simulink model "PV_MPPT (1)"  (R2025b)
settings: Solver=VariableStepAuto  StartTime=0.0  StopTime=160  FixedStep=0.01  MaxStep=1e-3  MinStep=1e-12  RelTol=1e-2
undefined symbols (not defined in the file): DiscIntNeverNeededParam
libraries: simulink x3, slpidlib x2

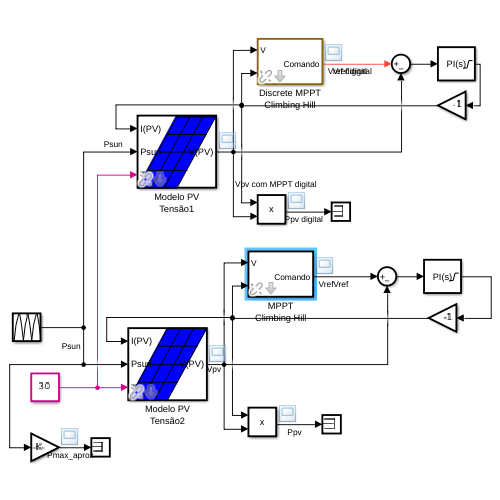
[thumbnail: Simulink's stored preview of the top-level diagram]
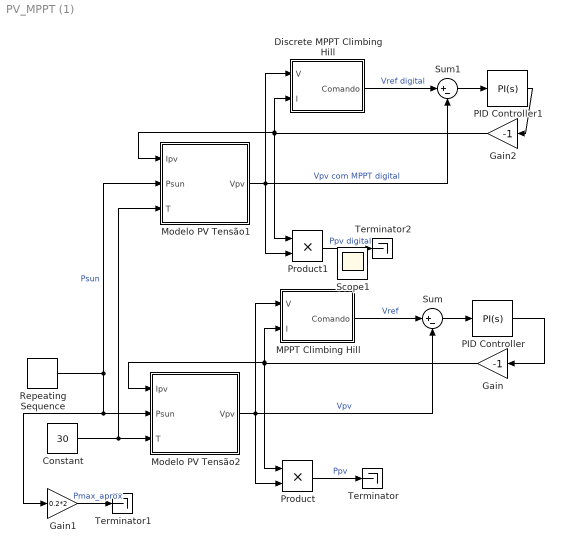
== system PV_MPPT (1) ==
  Constant : Constant  Value=30
  Discrete MPPT Climbing Hill : Subsystem  AncestorBlock=AvgModels/MPPT/MPPT Climbing Hill  mask(MPPT Hill Climbing){Ts=0.01, Passo=2, limsup=30*2, liminf=10*2, Inicial=25*2, sentido=Direto}
      mask prompts: Ts "Tempo de amostragem:"; Passo "Passo de variação"; limsup "Limite superior da saída:"; liminf "Limite inferior da saída:"; Inicial "Valor inicial:"; sentido "Direção do Comando:"
      mask help:
      | Algoritmo de rastreamento do ponto de máxima potência (MPPT).
      | Princípio da escalada ou Perturbe and Observe (P&O).
  Gain : Gain  Gain=-1
  Gain1 : Gain  Gain=0.2*2
  Gain2 : Gain  Gain=-1
  MPPT Climbing Hill : Subsystem  AncestorBlock=AvgModels/MPPT/MPPT Climbing Hill  mask(MPPT Hill Climbing){fb=100, Passo=2, limsup=30*2, liminf=15*2, Inicial=25*2, sentido=Direto}
      mask prompts: fb "Filtro de derivação:"; Passo "Passo de variação"; limsup "Limite superior da saída:"; liminf "Limite inferior da saída:"; Inicial "Valor inicial:"; sentido "Direção do comando:"
      mask help:
      | Algoritmo de rastreamento do ponto de máxima potência (MPPT).
      | Princípio da escalada ou Perturbe and Observe (P&O).
  Modelo PV Tensão1 : Subsystem  AncestorBlock=AvgModels/Fontes/Modelo PV Tensão  mask(Modelo PV de tensão){Ns=54, Voc=0.6093, Isc=8.21, Rs=0.005, Rp=7, Ms=2, Mp=1, Tr=273 + 25, a=3.18e-3, n=1.2, k=1.38e-23, q=1.60e-19, EG=1.1, tau=0.1, Psun=1000, Animar=off}
      mask prompts: Ns "Número de células"; Voc "Tensão de circuito aberto (Voc por célula)"; Isc "Corrente de curto-circuito (Isc)"; Rs "Resistência série da célula"; Rp "Resistência paralela da célula"; Ms "Módulos em Série"; Mp "Módulos em Paralelo"; Tr "Temperatura Ambiente (K)"; a "Coeficiente de temperatura de Isc:"; n "Fator de qualidade da junção p-n:"; k "Constante de Boltzmann:"; q "Carga do elétron:"; EG "Energia da banda proibida:"; tau "Contante de tempo (s):"; Psun "Irradiação de teste (W/m2):"; Animar "Animar em execução?"
      mask help:
      | Este é um modelo de tensão para painéis fotovoltaicos (sozinhos ou em arranjo).
      |
      | Fornece a tensão esperada de acordo com a corrente, a densidade de potência do sol e a temperatura ambiente.
      |
      | I(PV) é a corrente do arranjo fotovoltaico em Amperes.
      | Psun é a densidade de potência do sol em W/m2.
      | T é a temperatura ambiente em ºC.
      |
      | V(PV) é a tensão do arranjo fotovoltaico em Amperes.
      mask DialogControl ParameterGroupVar Prompt: Parâmetros
      mask DialogControl Container4 Prompt: Por módulo
      mask DialogControl Container6 Prompt: Local
      mask DialogControl Container5 Prompt: Constantes
      mask DialogControl Container9 Prompt: Verificação da curva.
      mask DialogControl Control2 Prompt: Verificar Curvas
      mask DialogControl Control2 Callback:
      | Psun = str2num(get_param(gcbh,'Psun'));
      | Tr = str2num(get_param(gcbh,'Tr'));
      | Voc = str2num(get_param(gcbh,'Voc'));
      | Isc = str2num(get_param(gcbh,'Isc'));
      | Rp = str2num(get_param(gcbh,'Rp'));
      | Rs = str2num(get_param(gcbh,'Rs'));
      | Ns = str2num(get_param(gcbh,'Ns'));
      | alpha = str2num(get_param(gcbh,'a'));
      | encontrapmax(Psun,Tr-273,Voc,Isc,Rp,Rs,Ns,alpha);
      mask Display:
      | % desenho detalhado
      | patch([0 .5 1 .5],[0 1 1 0],[0 0 1]);
      | plot([0 0.5],[0 1])
      | plot([0.5/3 0.5+0.5/3],[0 1])
      | plot([0.5/3 0.5+0.5/3]+0.5/3,[0 1])
      | plot([0.5 1],[0 1])
      | 
      | plot([0 0.5],[0 0])
      | plot([0 0.5]+0.125,[0 0]+0.25)
      | plot([0 0.5]+0.25,[0 0]+0.5)
      | plot([0 0.5]+0.25+0.125,[0 0]+0.75)
      | plot([0.5 1],[1 1])
      | 
      | 
      | port_label('output',1,'V(PV)');
      | 
      | port_label('input',1,'I(PV)');
      | port_label('input',2,'Psun');
      | port_label('input',3,'T');
  Modelo PV Tensão2 : Subsystem  AncestorBlock=AvgModels/Fontes/Modelo PV Tensão  mask(Modelo PV de tensão){Ns=54, Voc=0.6093, Isc=8.21, Rs=0.005, Rp=7, Ms=2, Mp=1, Tr=273 + 25, a=3.18e-3, n=1.2, k=1.38e-23, q=1.60e-19, EG=1.1, tau=0.1, Psun=1000, Animar=off}
      mask prompts: Ns "Número de células"; Voc "Tensão de circuito aberto (Voc por célula)"; Isc "Corrente de curto-circuito (Isc)"; Rs "Resistência série da célula"; Rp "Resistência paralela da célula"; Ms "Módulos em Série"; Mp "Módulos em Paralelo"; Tr "Temperatura Ambiente (K)"; a "Coeficiente de temperatura de Isc:"; n "Fator de qualidade da junção p-n:"; k "Constante de Boltzmann:"; q "Carga do elétron:"; EG "Energia da banda proibida:"; tau "Contante de tempo (s):"; Psun "Irradiação de teste (W/m2):"; Animar "Animar em execução?"
      mask help:
      | Este é um modelo de tensão para painéis fotovoltaicos (sozinhos ou em arranjo).
      |
      | Fornece a tensão esperada de acordo com a corrente, a densidade de potência do sol e a temperatura ambiente.
      |
      | I(PV) é a corrente do arranjo fotovoltaico em Amperes.
      | Psun é a densidade de potência do sol em W/m2.
      | T é a temperatura ambiente em ºC.
      |
      | V(PV) é a tensão do arranjo fotovoltaico em Amperes.
      mask DialogControl ParameterGroupVar Prompt: Parâmetros
      mask DialogControl Container4 Prompt: Por módulo
      mask DialogControl Container6 Prompt: Local
      mask DialogControl Container5 Prompt: Constantes
      mask DialogControl Container9 Prompt: Verificação da curva.
      mask DialogControl Control2 Prompt: Verificar Curvas
      mask DialogControl Control2 Callback:
      | Psun = str2num(get_param(gcbh,'Psun'));
      | Tr = str2num(get_param(gcbh,'Tr'));
      | Voc = str2num(get_param(gcbh,'Voc'));
      | Isc = str2num(get_param(gcbh,'Isc'));
      | Rp = str2num(get_param(gcbh,'Rp'));
      | Rs = str2num(get_param(gcbh,'Rs'));
      | Ns = str2num(get_param(gcbh,'Ns'));
      | alpha = str2num(get_param(gcbh,'a'));
      | encontrapmax(Psun,Tr-273,Voc,Isc,Rp,Rs,Ns,alpha);
      mask Display:
      | % desenho detalhado
      | patch([0 .5 1 .5],[0 1 1 0],[0 0 1]);
      | plot([0 0.5],[0 1])
      | plot([0.5/3 0.5+0.5/3],[0 1])
      | plot([0.5/3 0.5+0.5/3]+0.5/3,[0 1])
      | plot([0.5 1],[0 1])
      | 
      | plot([0 0.5],[0 0])
      | plot([0 0.5]+0.125,[0 0]+0.25)
      | plot([0 0.5]+0.25,[0 0]+0.5)
      | plot([0 0.5]+0.25+0.125,[0 0]+0.75)
      | plot([0.5 1],[1 1])
      | 
      | 
      | port_label('output',1,'V(PV)');
      | 
      | port_label('input',1,'I(PV)');
      | port_label('input',2,'Psun');
      | port_label('input',3,'T');
  PID Controller : slpidlib/PID Controller  Controller=PI  Form=Parallel  TimeDomain=Continuous-time  UseExternalTs=off  SampleTime=-1  IntegratorMethod=Forward Euler  FilterMethod=Forward Euler  ControllerParametersSource=internal  P=1  I=1  UseKiTs=off  D=0  UseExternalDerivativeSource=off  N=100  UseFilter=on  TunerSelectOption=Transfer Function Based (PID Tuner App)  InitialConditionSource=internal  InitialConditionForIntegrator=-1  InitialConditionForFilter=0  DifferentiatorICPrevScaledInput=0  ExternalReset=none  TrackingMode=off  Kt=1  LimitOutput=on  SatLimitsSource=internal  UpperSaturationLimit=-0.5  LowerSaturationLimit=-8  LinearizeAsGain=on  AntiWindupMode=none  Kb=1  LimitIntegrator=off  UpperIntegratorSaturationLimit=inf  LowerIntegratorSaturationLimit=-inf  POutMin=[]  POutMax=[]  IOutMin=[]  IOutMax=[]  DOutMin=[]  DOutMax=[]  NOutMin=[]  NOutMax=[]  SumOutMin=[]  SumOutMax=[]  SaturationOutMin=[]  SaturationOutMax=[]  PParamMin=[]  PParamMax=[]  IParamMin=[]  IParamMax=[]  DParamMin=[]  DParamMax=[]  NParamMin=[]  NParamMax=[]  KbParamMin=[]  KbParamMax=[]  KtParamMin=[]  KtParamMax=[]  KbOutMin=[]  KbOutMax=[]  KtOutMin=[]  KtOutMax=[]  IntegratorOutMin=[]  IntegratorOutMax=[]  FilterOutMin=[]  FilterOutMax=[]  SumI1OutMin=[]  SumI1OutMax=[]  SumI2OutMin=[]  SumI2OutMax=[]  SumI3OutMin=[]  SumI3OutMax=[]  SumI4OutMin=[]  SumI4OutMax=[]  SumDOutMin=[]  SumDOutMax=[]  DifferentiatorOutMin=[]  DifferentiatorOutMax=[]  FilterDiffOutCoefMin=[]  FilterDiffOutCoefMax=[]  ReciprocalOutMin=[]  ReciprocalOutMax=[]  SumDenOutMin=[]  SumDenOutMax=[]  SumNumOutMin=[]  SumNumOutMax=[]  DivideOutMin=[]  DivideOutMax=[]  UdiffTsProdOutMin=[]  UdiffTsProdOutMax=[]  NTsProdOutMin=[]  NTsProdOutMax=[]  UintegralTsProdOutMin=[]  UintegralTsProdOutMax=[]  UngainTsProdOutMin=[]  UngainTsProdOutMax=[]  ClampingZeroOutDataTypeStr=Inherit: Inherit via back propagation  ClampingZeroOutMin=[]  ClampingZeroOutMax=[]  FilterDenConstantOutDataTypeStr=Inherit: Inherit via back propagation  FilterDenConstantOutMin=[]  FilterDenConstantOutMax=[]  PCopyOutDataTypeStr=Inherit: Inherit via back propagation  PCopyOutMin=[]  PCopyOutMax=[]  NCopyOutDataTypeStr=Inherit: Inherit via back propagation  NCopyOutMin=[]  NCopyOutMax=[]  IntegratorContinuousStateAttributes=''  IntegratorStateMustResolveToSignalObject=off  IntegratorRTWStateStorageClass=Auto  FilterContinuousStateAttributes=''  FilterStateMustResolveToSignalObject=off  FilterRTWStateStorageClass=Auto  ParallelPVariant=InternalParameters  IdealPVariant=Disabled  IVariant=InternalParameters  DVariant=Disabled  IntegratorVariant=Continuous  SatVariant=Enabled  AWVariant=Passthrough  PCopyVariant=Disabled  TRVariant=Disabled  FdbkBlocksVariant=Forward  IdealPFdbkVariant=Disabled  SatFdbkVariant=Disabled  DerivativeFilterVariant=Disabled  NVariant=Disabled  NCopyVariant=Disabled_SignalSpec  FilterICVariant=Disabled  IntegratorICVariant=InternalICs  ExternalResetVariant=Disabled  TRSumVariant=Passthrough  SumFdbkVariant=Disabled  SumVariant=Sum_PI  TsampFilterVariant=InternalTs  TsampNgainVariant=Passthrough  TsampIntegralVariant=Disabled_SignalSpec  ExternalSaturationOutDataTypeStr=Inherit: Same as second input  DerivativeSourceVariant=Disabled  PreIntVariant=InternalPreInt
  PID Controller1 : slpidlib/PID Controller  Controller=PI  Form=Parallel  TimeDomain=Continuous-time  UseExternalTs=off  SampleTime=-1  IntegratorMethod=Forward Euler  FilterMethod=Forward Euler  ControllerParametersSource=internal  P=1  I=1  UseKiTs=off  D=0  UseExternalDerivativeSource=off  N=100  UseFilter=on  TunerSelectOption=Transfer Function Based (PID Tuner App)  InitialConditionSource=internal  InitialConditionForIntegrator=-1  InitialConditionForFilter=0  DifferentiatorICPrevScaledInput=0  ExternalReset=none  TrackingMode=off  Kt=1  LimitOutput=on  SatLimitsSource=internal  UpperSaturationLimit=-0.5  LowerSaturationLimit=-8  LinearizeAsGain=on  AntiWindupMode=clamping  Kb=1  LimitIntegrator=off  UpperIntegratorSaturationLimit=inf  LowerIntegratorSaturationLimit=-inf  POutMin=[]  POutMax=[]  IOutMin=[]  IOutMax=[]  DOutMin=[]  DOutMax=[]  NOutMin=[]  NOutMax=[]  SumOutMin=[]  SumOutMax=[]  SaturationOutMin=[]  SaturationOutMax=[]  PParamMin=[]  PParamMax=[]  IParamMin=[]  IParamMax=[]  DParamMin=[]  DParamMax=[]  NParamMin=[]  NParamMax=[]  KbParamMin=[]  KbParamMax=[]  KtParamMin=[]  KtParamMax=[]  KbOutMin=[]  KbOutMax=[]  KtOutMin=[]  KtOutMax=[]  IntegratorOutMin=[]  IntegratorOutMax=[]  FilterOutMin=[]  FilterOutMax=[]  SumI1OutMin=[]  SumI1OutMax=[]  SumI2OutMin=[]  SumI2OutMax=[]  SumI3OutMin=[]  SumI3OutMax=[]  SumI4OutMin=[]  SumI4OutMax=[]  SumDOutMin=[]  SumDOutMax=[]  DifferentiatorOutMin=[]  DifferentiatorOutMax=[]  FilterDiffOutCoefMin=[]  FilterDiffOutCoefMax=[]  ReciprocalOutMin=[]  ReciprocalOutMax=[]  SumDenOutMin=[]  SumDenOutMax=[]  SumNumOutMin=[]  SumNumOutMax=[]  DivideOutMin=[]  DivideOutMax=[]  UdiffTsProdOutMin=[]  UdiffTsProdOutMax=[]  NTsProdOutMin=[]  NTsProdOutMax=[]  UintegralTsProdOutMin=[]  UintegralTsProdOutMax=[]  UngainTsProdOutMin=[]  UngainTsProdOutMax=[]  ClampingZeroOutDataTypeStr=Inherit: Inherit via back propagation  ClampingZeroOutMin=[]  ClampingZeroOutMax=[]  FilterDenConstantOutDataTypeStr=Inherit: Inherit via back propagation  FilterDenConstantOutMin=[]  FilterDenConstantOutMax=[]  PCopyOutDataTypeStr=Inherit: Inherit via back propagation  PCopyOutMin=[]  PCopyOutMax=[]  NCopyOutDataTypeStr=Inherit: Inherit via back propagation  NCopyOutMin=[]  NCopyOutMax=[]  IntegratorContinuousStateAttributes=''  IntegratorStateMustResolveToSignalObject=off  IntegratorRTWStateStorageClass=Auto  FilterContinuousStateAttributes=''  FilterStateMustResolveToSignalObject=off  FilterRTWStateStorageClass=Auto  ParallelPVariant=InternalParameters  IdealPVariant=Disabled  IVariant=InternalParameters  DVariant=Disabled  IntegratorVariant=Continuous  SatVariant=Enabled  AWVariant=ContClampingParallel  PCopyVariant=Disabled  TRVariant=Disabled  FdbkBlocksVariant=Forward  IdealPFdbkVariant=Disabled  SatFdbkVariant=Disabled  DerivativeFilterVariant=Disabled  NVariant=Disabled  NCopyVariant=Disabled_SignalSpec  FilterICVariant=Disabled  IntegratorICVariant=InternalICs  ExternalResetVariant=Disabled  TRSumVariant=Passthrough  SumFdbkVariant=Disabled  SumVariant=Sum_PI  TsampFilterVariant=InternalTs  TsampNgainVariant=Passthrough  TsampIntegralVariant=Disabled_SignalSpec  ExternalSaturationOutDataTypeStr=Inherit: Same as second input  DerivativeSourceVariant=Disabled  PreIntVariant=InternalPreInt
  Product : Product
  Product1 : Product
  Repeating Sequence : simulink/Sources/Repeating Sequence  rep_seq_t=[0 2 4 5 6 8 10]*4  rep_seq_y=[1 5 7 8 8 5 1]*100
  Sum : Sum  Inputs=|+-
  Sum1 : Sum  Inputs=|+-
  Terminator : Terminator
  Terminator1 : Terminator
  Terminator2 : Terminator
  Scope1 : Scope
      settings: ActiveDisplayYMinimum=-7.8557532744699214  ActiveDisplayYMaximum=70.701779470229312
  wires:
  Modelo PV Tensão2/1(Vpv) -> Sum/2, Product/2, MPPT Climbing Hill/1(V)  "Vpv"
  Sum/1 -> PID Controller/1
  PID Controller/1 -> Gain/1
  Gain/1 -> Modelo PV Tensão2/1(Ipv), MPPT Climbing Hill/2(I), Product/1
  Product/1 -> Terminator/1  "Ppv"
  Gain1/1 -> Terminator1/1  "Pmax_aprox"
  MPPT Climbing Hill/1(Comando) -> Sum/1  "Vref"
  Discrete MPPT Climbing Hill/1(Comando) -> Sum1/1  "Vref digital"
  Product1/1 -> Terminator2/1  "Ppv digital"
  Gain2/1 -> Product1/1, Discrete MPPT Climbing Hill/2(I), Modelo PV Tensão1/1(Ipv)
  PID Controller1/1 -> Gain2/1
  Repeating Sequence/1 -> Modelo PV Tensão2/2(Psun), Gain1/1, Modelo PV Tensão1/2(Psun)  "Psun"
  Constant/1 -> Modelo PV Tensão2/3(T), Modelo PV Tensão1/3(T)
  Sum1/1 -> PID Controller1/1
  Modelo PV Tensão1/1(Vpv) -> Discrete MPPT Climbing Hill/1(V), Product1/2, Sum1/2  "Vpv com MPPT digital"

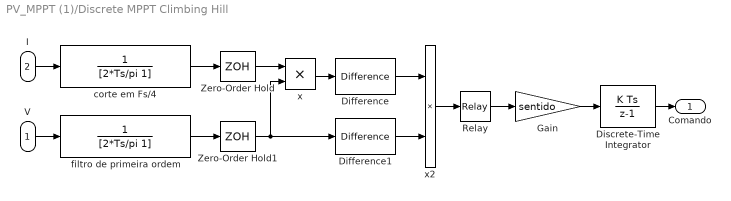
== system PV_MPPT (1)/Discrete MPPT Climbing Hill ==
  V : Inport
  I : Inport  Port=2
  Difference : simulink/Discrete/Difference  ICPrevInput=Ts  OutMin=[]  OutMax=[]  OutDataType=fixdt(1, 16)  OutScaling=2^-10  DoSatur=off
  Difference1 : simulink/Discrete/Difference  ICPrevInput=Ts  OutMin=[]  OutMax=[]  OutDataType=fixdt(1, 16)  OutScaling=2^-10  DoSatur=off
  Discrete-Time Integrator : DiscreteIntegrator  gainval=Passo  InitialCondition=Inicial  SampleTime=Ts  LimitOutput=on  UpperSaturationLimit=limsup  LowerSaturationLimit=liminf  ICPrevOutput=DiscIntNeverNeededParam  ICPrevScaledInput=DiscIntNeverNeededParam
  Gain : Gain  Gain=sentido
  Relay : Relay  OnSwitchValue=1  OffSwitchValue=-1  OffOutputValue=-1  ZeroCross=off
  Zero-Order Hold : ZeroOrderHold  SampleTime=Ts
  Zero-Order Hold1 : ZeroOrderHold  SampleTime=Ts
  corte em Fs/4 : TransferFcn  Denominator=[2*Ts/pi 1]
  filtro de primeira ordem : TransferFcn  Denominator=[2*Ts/pi 1]
  x : Product  RndMeth=Zero
  x2 : Product  RndMeth=Zero
  Comando : Outport
  wires:
  x/1 -> Difference/1
  Difference/1 -> x2/1
  Difference1/1 -> x2/2
  V/1 -> filtro de primeira ordem/1
  I/1 -> corte em Fs/4/1
  x2/1 -> Relay/1
  Relay/1 -> Gain/1
  Discrete-Time Integrator/1 -> Comando/1
  Zero-Order Hold/1 -> x/1
  Zero-Order Hold1/1 -> x/2, Difference1/1
  corte em Fs/4/1 -> Zero-Order Hold/1
  filtro de primeira ordem/1 -> Zero-Order Hold1/1
  Gain/1 -> Discrete-Time Integrator/1

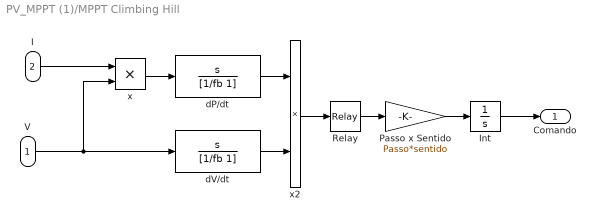
== system PV_MPPT (1)/MPPT Climbing Hill ==
  V : Inport
  I : Inport  Port=2
  Int : Integrator  InitialCondition=Inicial  LimitOutput=on  UpperSaturationLimit=limsup  LowerSaturationLimit=liminf
  Passo x Sentido : Gain  Gain=Passo*sentido
  Relay : Relay  OnSwitchValue=1  OffSwitchValue=-1  OffOutputValue=-1  ZeroCross=off
  dP/dt : TransferFcn  Numerator=[1 0]  Denominator=[1/fb 1]
  dV/dt : TransferFcn  Numerator=[1 0]  Denominator=[1/fb 1]
  x : Product  RndMeth=Zero
  x2 : Product  RndMeth=Zero
  Comando : Outport
  wires:
  Int/1 -> Comando/1
  x2/1 -> Relay/1
  I/1 -> x/1
  V/1 -> x/2, dV/dt/1
  dV/dt/1 -> x2/2
  dP/dt/1 -> x2/1
  x/1 -> dP/dt/1
  Relay/1 -> Passo x Sentido/1
  Passo x Sentido/1 -> Int/1

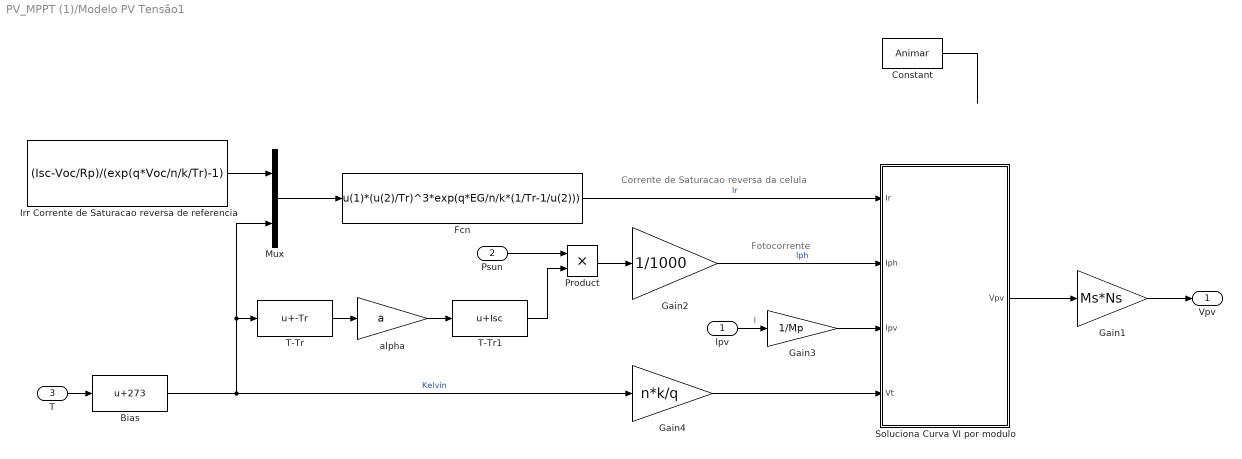
== system PV_MPPT (1)/Modelo PV Tensão1 ==
  note: Fotocorrente
  note: Corrente de Saturacao reversa da celula
  Ipv : Inport
  Psun : Inport  Port=2
  T : Inport  Port=3
  Bias : Bias  Bias=273  SaturateOnIntegerOverflow=off
  Constant : Constant  Value=Animar
  Fcn : Fcn  Expr=u(1)*(u(2)/Tr)^3*exp(q*EG/n/k*(1/Tr-1/u(2)))
  Gain1 : Gain  Gain=Ms*Ns
  Gain2 : Gain  Gain=1/1000
  Gain3 : Gain  Gain=1/Mp
  Gain4 : Gain  Gain=n*k/q
  Irr Corrente de Saturacao reversa de referencia : Constant  Value=(Isc-Voc/Rp)/(exp(q*Voc/n/k/Tr)-1)
  Mux : Mux  Inputs=2
  Product : Product
  Soluciona Curva VI por modulo : Subsystem
  T-Tr : Bias  Bias=-Tr  SaturateOnIntegerOverflow=off
  T-Tr1 : Bias  Bias=Isc  SaturateOnIntegerOverflow=off
  alpha : Gain  Gain=a
  Vpv : Outport
  wires:
  Irr Corrente de Saturacao reversa de referencia/1 -> Mux/1
  Mux/1 -> Fcn/1
  Psun/1 -> Product/1
  T-Tr1/1 -> Product/2
  Product/1 -> Gain2/1
  alpha/1 -> T-Tr1/1
  T-Tr/1 -> alpha/1
  T/1 -> Bias/1
  Bias/1 -> T-Tr/1, Mux/2, Gain4/1  "Kelvin"
  Gain4/1 -> Soluciona Curva VI por modulo/4(Vt)
  Fcn/1 -> Soluciona Curva VI por modulo/1(Ir)  "Ir"
  Gain2/1 -> Soluciona Curva VI por modulo/2(Iph)  "Iph"
  Ipv/1 -> Gain3/1  "I"
  Soluciona Curva VI por modulo/1(Vpv) -> Gain1/1
  Gain1/1 -> Vpv/1
  Gain3/1 -> Soluciona Curva VI por modulo/3(Ipv)
  Constant/1 -> ?

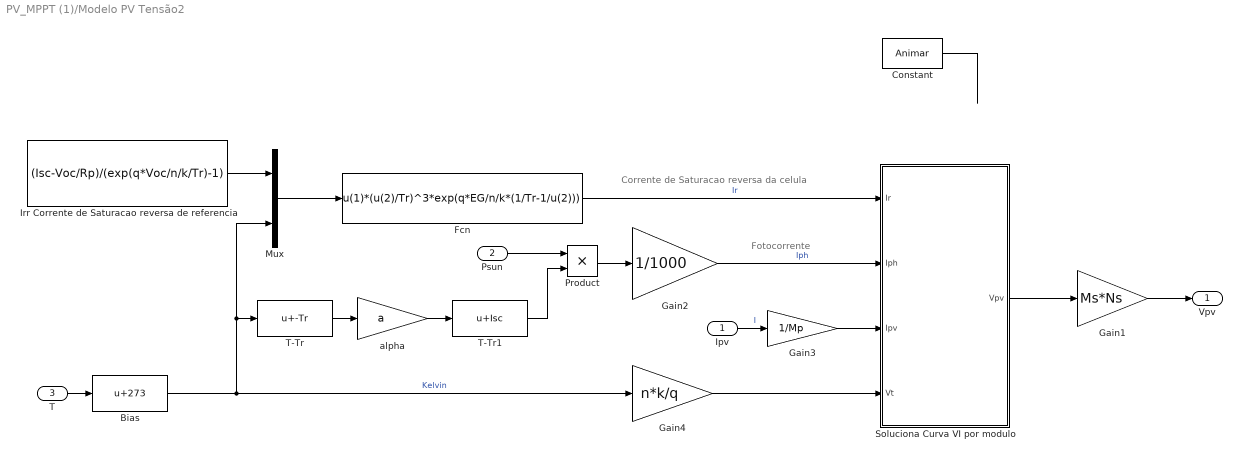
== system PV_MPPT (1)/Modelo PV Tensão2 ==
  note: Corrente de Saturacao reversa da celula
  note: Fotocorrente
  Ipv : Inport
  Psun : Inport  Port=2
  T : Inport  Port=3
  Bias : Bias  Bias=273  SaturateOnIntegerOverflow=off
  Constant : Constant  Value=Animar
  Fcn : Fcn  Expr=u(1)*(u(2)/Tr)^3*exp(q*EG/n/k*(1/Tr-1/u(2)))
  Gain1 : Gain  Gain=Ms*Ns
  Gain2 : Gain  Gain=1/1000
  Gain3 : Gain  Gain=1/Mp
  Gain4 : Gain  Gain=n*k/q
  Irr Corrente de Saturacao reversa de referencia : Constant  Value=(Isc-Voc/Rp)/(exp(q*Voc/n/k/Tr)-1)
  Mux : Mux  Inputs=2
  Product : Product
  Soluciona Curva VI por modulo : Subsystem
  T-Tr : Bias  Bias=-Tr  SaturateOnIntegerOverflow=off
  T-Tr1 : Bias  Bias=Isc  SaturateOnIntegerOverflow=off
  alpha : Gain  Gain=a
  Vpv : Outport
  wires:
  Constant/1 -> ?
  Gain3/1 -> Soluciona Curva VI por modulo/3(Ipv)
  Gain1/1 -> Vpv/1
  Soluciona Curva VI por modulo/1(Vpv) -> Gain1/1
  Ipv/1 -> Gain3/1  "I"
  Gain2/1 -> Soluciona Curva VI por modulo/2(Iph)  "Iph"
  Fcn/1 -> Soluciona Curva VI por modulo/1(Ir)  "Ir"
  Gain4/1 -> Soluciona Curva VI por modulo/4(Vt)
  Bias/1 -> Gain4/1, Mux/2, T-Tr/1  "Kelvin"
  T/1 -> Bias/1
  T-Tr/1 -> alpha/1
  alpha/1 -> T-Tr1/1
  Product/1 -> Gain2/1
  T-Tr1/1 -> Product/2
  Psun/1 -> Product/1
  Mux/1 -> Fcn/1
  Irr Corrente de Saturacao reversa de referencia/1 -> Mux/1

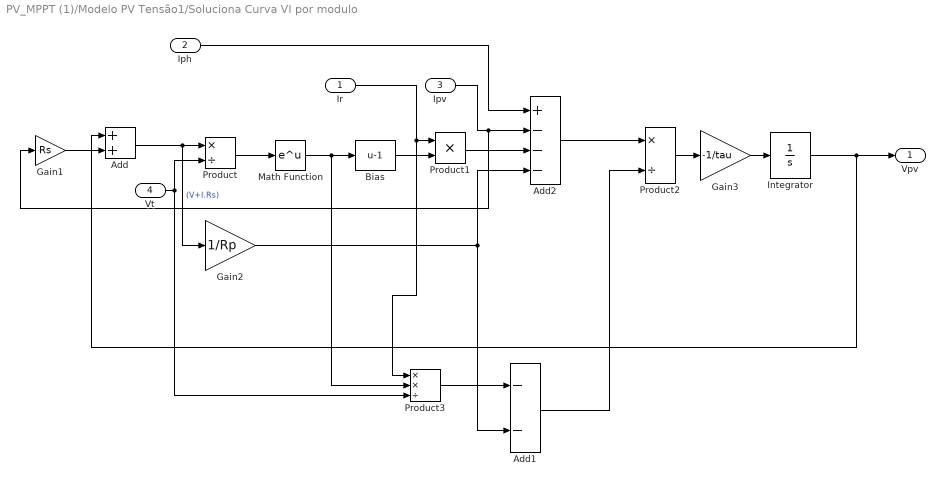
== system PV_MPPT (1)/Modelo PV Tensão1/Soluciona Curva VI por modulo ==
  Ir : Inport
  Iph : Inport  Port=2
  Ipv : Inport  Port=3
  Vt : Inport  Port=4
  Add : Sum
  Add1 : Sum  Inputs=--
  Add2 : Sum  Inputs=+---
  Bias : Bias  Bias=-1  SaturateOnIntegerOverflow=off
  Gain1 : Gain  Gain=Rs
  Gain2 : Gain  Gain=1/Rp
  Gain3 : Gain  Gain=-1/tau
  Integrator : Integrator  LimitOutput=on  LowerSaturationLimit=0
  Math Function : Math  SignedPower=on
  Product : Product  Inputs=*/
  Product1 : Product
  Product2 : Product  Inputs=*/
  Product3 : Product  Inputs=**/
  Vpv : Outport
  wires:
  Ipv/1 -> Gain1/1, Add2/2
  Add2/1 -> Product2/1
  Product1/1 -> Add2/3
  Iph/1 -> Add2/1
  Ir/1 -> Product3/1, Product1/1
  Bias/1 -> Product1/2
  Math Function/1 -> Product3/2, Bias/1
  Product/1 -> Math Function/1
  Add/1 -> Product/1, Gain2/1  "(V+I.Rs)"
  Vt/1 -> Product3/3, Product/2
  Integrator/1 -> Vpv/1, Add/1
  Gain1/1 -> Add/2
  Product2/1 -> Gain3/1
  Product3/1 -> Add1/1
  Gain2/1 -> Add2/4, Add1/2
  Add1/1 -> Product2/2
  Gain3/1 -> Integrator/1

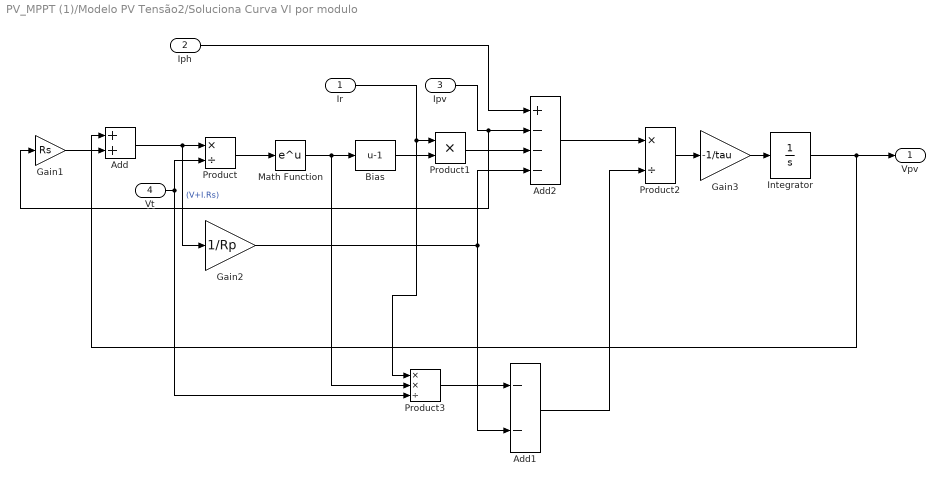
== system PV_MPPT (1)/Modelo PV Tensão2/Soluciona Curva VI por modulo ==
  Ir : Inport
  Iph : Inport  Port=2
  Ipv : Inport  Port=3
  Vt : Inport  Port=4
  Add : Sum
  Add1 : Sum  Inputs=--
  Add2 : Sum  Inputs=+---
  Bias : Bias  Bias=-1  SaturateOnIntegerOverflow=off
  Gain1 : Gain  Gain=Rs
  Gain2 : Gain  Gain=1/Rp
  Gain3 : Gain  Gain=-1/tau
  Integrator : Integrator  LimitOutput=on  LowerSaturationLimit=0
  Math Function : Math  SignedPower=on
  Product : Product  Inputs=*/
  Product1 : Product
  Product2 : Product  Inputs=*/
  Product3 : Product  Inputs=**/
  Vpv : Outport
  wires:
  Gain3/1 -> Integrator/1
  Add1/1 -> Product2/2
  Gain2/1 -> Add1/2, Add2/4
  Product3/1 -> Add1/1
  Product2/1 -> Gain3/1
  Gain1/1 -> Add/2
  Integrator/1 -> Add/1, Vpv/1
  Vt/1 -> Product/2, Product3/3
  Add/1 -> Gain2/1, Product/1  "(V+I.Rs)"
  Product/1 -> Math Function/1
  Math Function/1 -> Bias/1, Product3/2
  Bias/1 -> Product1/2
  Ir/1 -> Product1/1, Product3/1
  Iph/1 -> Add2/1
  Product1/1 -> Add2/3
  Add2/1 -> Product2/1
  Ipv/1 -> Add2/2, Gain1/1
